simulink model "M10B39"  (R2025a)
settings: Solver=ode23tb  StartTime=0.0  StopTime=20  FixedStep=0.001  MaxStep=0.01  RelTol=1e-3  EnableMultiTasking=on
InitFcn:
  | initAll
values from neighbouring files (symbols this model uses):
  acom = 100    [initAll.m]    (also in initAll_V2.m)
  bcom = 50    [initAll.m]    (also in initAll_V2.m)
  commun = 0*commun    [initAll.m]    (also in initAll_V2.m)
  DataDelay = 0.0*DataDelay    [initAll.m]    (also in initAll_V2.m)
  fB = 50    [initAll.m]    (also in initAll_V2.m)
  Geninit = Generator_init(opdata,SynMach_in_gidx)    [initAll.m]    (also in initAll_V2.m)
  lam = 100    [initAll.m]    (also in initAll_V2.m)
  SgridB = 100    [initAll.m]    (also in initAll_V2.m)
  wB = 2*pi*fB    (= 314.159265359)    [initAll.m]    (also in initAll_V2.m)
undefined symbols (not defined in the file or in its folder): AVm0, c1, c2, c3, c4, c5, c6, cp_nom, ESinit, lambda_nom, P_wind_base, Pelec_base, Pnom, Windinit, YY_load
libraries: spsBistableLib x10, simulink_extras x6, simulink x1
(part 1 of 8)
settings Model: Creator=m  LastModifiedBy=86182
settings SolverCC: AlgebraicLoopSolver=TrustRegion
settings DataIOCC: LimitDataPoints=on  SaveFormat=Array  SignalLoggingSaveFormat=ModelDataLogs  ReturnWorkspaceOutputs=off  SignalLoggingName=sigsOut
settings OptimizationCC: ExpressionDepthLimit=2147483647.0  LifeSpan=inf
settings DebuggingCC: SaveWithParameterizedLinksMsg=none  UnderspecifiedInitializationDetection=Classic  MergeDetectMultiDrivingBlocksExec=none  SignalResolutionControl=TryResolveAllWithWarning  MultiTaskDSMMsg=warning  MultiTaskCondExecSysMsg=none  FcnCallInpInsideContextMsg=warning  UnconnectedInputMsg=warning  UnconnectedOutputMsg=warning  UnconnectedLineMsg=warning  StateNameClashWarn=warning  SFUnexpectedBacktrackingDiag=warning  SFNoUnconditionalDefaultTransitionDiag=warning  SFExecutionAtInitializationDiag=none  ArithmeticOperatorsInVariantConditions=warning
settings HardwareCC: ProdBitPerPointer=32.0  ProdBitPerSizeT=32.0  ProdBitPerPtrDiffT=32.0  ProdLargestAtomicFloat=None  ProdIntDivRoundTo=Undefined  ProdEndianess=Unspecified  ProdWordSize=32.0  ProdHWDeviceType=32-bit Generic  TargetUnknown=on
settings ModelReferenceCC: EnableRefExpFcnMdlSchedulingChecks=on  PropagateSignalLabelsOutOfModel=off
settings SFSimCC: SimUseLocalCustomCode=off  CustomCodeUndefinedFunction=UseInterfaceOnly
settings RTWCC: RTWUseLocalCustomCode=off  GPUComputeCapability=3.5
settings CodeAppCC: StateflowObjectComments=on
settings GRTTargetCC: TargetLangStandard=C89/C90 (ANSI)  CombineOutputUpdateFcns=off  GRTInterface=on
settings ConfigComp: CovMetricSettings=dw  CovSaveCumulativeToWorkspaceVar=on  CovSaveSingleToWorkspaceVar=on  CovExternalEMLEnable=off  CovSFcnEnable=off

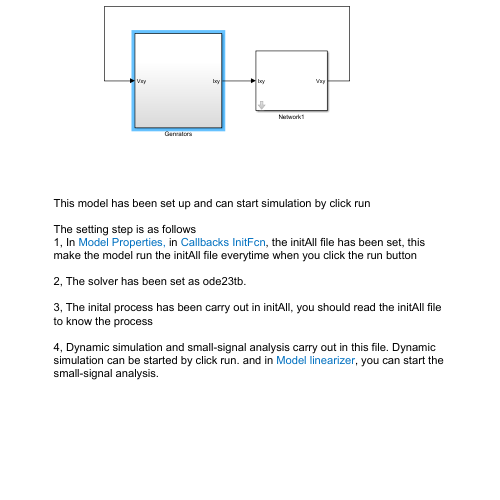
[thumbnail: Simulink's stored preview of the top-level diagram]
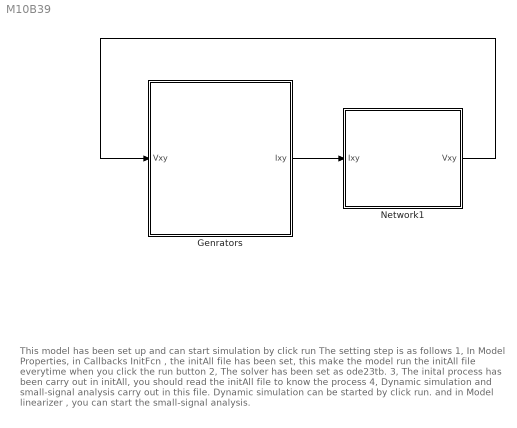
== system M10B39 ==
  note: This model has been set up and can start simulation by click run
      |
      | The setting step is as follows
      | 1, In Model Properties, in Callbacks InitFcn , the initAll file has been set, this make the model run the initAll file everytime when you click the run button
      |
      | 2, The solver has been set as ode23tb.
      |
      | 3, The inital process has been carry out in initAll, you should read the initAll file to know the process
      |
      | 4, Dynamic simulation and small-signal analysis carry out in this file. Dynamic simulation can be started by click run. and in Model linearizer , you can start the small-signal analysis.
  Genrators : Subsystem
  Network1 : Subsystem  mask{YY_load=YY_load, ng=10}
  wires:
  Genrators/1(Ixy) -> Network1/1(Ixy)
  Network1/1(Vxy) -> Genrators/1(Vxy)

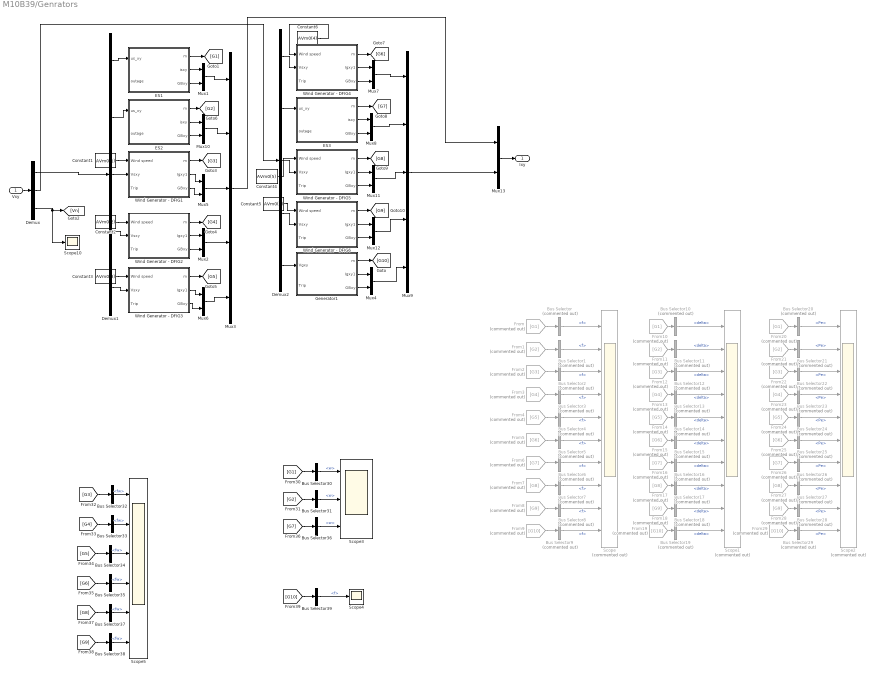
== system M10B39/Genrators ==
  Vxy : Inport
  Bus Selector{,1..9} (10 alike) : BusSelector  Commented=on  OutputSignals=f
  Bus Selector{10..19} (10 alike) : BusSelector  Commented=on  OutputSignals=delta
  Bus Selector{20..29} (10 alike) : BusSelector  Commented=on  OutputSignals=Pe
  Bus Selector30 : BusSelector  OutputSignals=w
  Bus Selector31 : BusSelector  OutputSignals=w
  Bus Selector{32..35,37..38} (6 alike) : BusSelector  OutputSignals=fw
  Bus Selector36 : BusSelector  OutputSignals=w
  Bus Selector39 : BusSelector  OutputSignals=f
  Constant1 : Constant  Value=AVm0(1)
  Constant2 : Constant  Value=AVm0(2)
  Constant3 : Constant  Value=AVm0(3)
  Constant4 : Constant  Value=AVm0(5)
  Constant5 : Constant  Value=AVm0(6)
  Constant6 : Constant  Value=AVm0(4)
  Demux : Demux  Outputs=[10 10 29]
      settings: DisplayOption=none
  Demux1 : Demux  Outputs=5
      settings: DisplayOption=none
  Demux2 : Demux  Outputs=5
      settings: DisplayOption=none
  ES1 : Subsystem  mask{SvscB=ESinit.SvscBi(1), SgridB=SgridB, Kppll_VSC=ESinit.Kppll(1), Kipll_VSC=ESinit.Kipll(1), Dels_hvdc=ESinit.Dels_hvdc(1), Lpr=ESinit.Lpr(1), Rpr=ESinit.Rpr(1), wB=wB, Is_xA_0=ESinit.Isx0(1), Is_yA_0=ESinit.Isy0(1), KpP_VSC_A=ESinit.KpP(1), KiP_VSC_A=ESinit.KiP(1), KpId_VSC_A=ESinit.KpId(1), KiId_VSC_A=ESinit.KiId(1), KpQ_VSC_A=ESinit.KpQ(1), KiQ_VSC_A=ESinit.KiQ(1), KpIq_VSC_A=ESinit.KpIq(1), KiIq_VSC_A=ESinit.KiIq(1), Md_A_0=ESinit.Md0(1), Mq_A_0=ESinit.Mq0(1), Nd_A_0=ESinit.Nd0(1), Nq_A_0=ESinit.Nq0(1), KIR=ESinit.Kir(1), Kdroop=ESinit.Kdroop(1), Kdistributed=ESinit.Kdistributed(1), Kdistributed_d=ESinit.Kdistributed_d(1), Kpac_VSC_A=ESinit.Kpac(1), Kiac_VSC_A=ESinit.Kiac(1), P0=ESinit.P0(1), Q0=ESinit.Q0(1), usd0=ESinit.Usd0(1)}
      mask prompts: Kppll_VSC "Kppll"; Kipll_VSC "Kipll"; KpP_VSC_A "KpP"; KiP_VSC_A "KiP"; KpId_VSC_A "KpId"; KiId_VSC_A "KiId"; KpQ_VSC_A "KpQ"; KiQ_VSC_A "KiQ"; KpIq_VSC_A "KpIq"; KiIq_VSC_A "KiIq"; Kpac_VSC_A "Kpac"; Kiac_VSC_A "Kiac"
      mask DialogControl Container48 Prompt: Base value
      mask DialogControl Container7 Prompt: PLL
      mask DialogControl Container5 Prompt: Control parameter
      mask DialogControl Container8 Prompt: inital value
      mask DialogControl Container9 Prompt: AC side
      mask DialogControl Container10 Prompt: Parameter
      mask DialogControl Container11 Prompt: Initial value
      mask DialogControl Container18 Prompt: Control parameter
      mask DialogControl Container19 Prompt: d_axis_control parameter
      mask DialogControl Container23 Prompt: d_axis_control=1
      mask DialogControl Container26 Prompt: inner current control
      mask DialogControl Container21 Prompt: q_axis_control parameter
      mask DialogControl Container29 Prompt: q_axis_control=1
      mask DialogControl Container31 Prompt: inner current control
      mask DialogControl Container22 Prompt: inital value
      mask DialogControl Container35 Prompt: outer controller
      mask DialogControl Container36 Prompt: inner control
      mask DialogControl Container27 Prompt: Inertia control
      mask DialogControl Container28 Prompt: droop control
      mask DialogControl Container300 Prompt: distributed control
      mask DialogControl Container301 Prompt: Droop distributed control
      mask DialogControl Container40 Prompt: usdq_control
      mask DialogControl Container41 Prompt: PQinitial
      mask DialogControl Container42 Prompt: usd0initial
  ES2 : Subsystem  mask{SvscB=ESinit.SvscBi(2), SgridB=SgridB, Kppll_VSC=ESinit.Kppll(2), Kipll_VSC=ESinit.Kipll(2), Dels_hvdc=ESinit.Dels_hvdc(2), Lpr=ESinit.Lpr(2), Rpr=ESinit.Rpr(2), wB=wB, Is_xA_0=ESinit.Isx0(2), Is_yA_0=ESinit.Isy0(2), KpP_VSC_A=ESinit.KpP(2), KiP_VSC_A=ESinit.KiP(2), KpId_VSC_A=ESinit.KpId(2), KiId_VSC_A=ESinit.KiId(2), KpQ_VSC_A=ESinit.KpQ(2), KiQ_VSC_A=ESinit.KiQ(2), KpIq_VSC_A=ESinit.KpIq(2), KiIq_VSC_A=ESinit.KiIq(2), Md_A_0=ESinit.Md0(2), Mq_A_0=ESinit.Mq0(2), Nd_A_0=ESinit.Nd0(2), Nq_A_0=ESinit.Nq0(2), KIR=ESinit.Kir(2), Kdroop=ESinit.Kdroop(2), Kdistributed=ESinit.Kdistributed(2), Kdistributed_d=ESinit.Kdistributed_d(2), Kpac_VSC_A=ESinit.Kpac(2), Kiac_VSC_A=ESinit.Kiac(2), P0=ESinit.P0(2), Q0=ESinit.Q0(2), usd0=ESinit.Usd0(2)}
      mask prompts: Kppll_VSC "Kppll"; Kipll_VSC "Kipll"; KpP_VSC_A "KpP"; KiP_VSC_A "KiP"; KpId_VSC_A "KpId"; KiId_VSC_A "KiId"; KpQ_VSC_A "KpQ"; KiQ_VSC_A "KiQ"; KpIq_VSC_A "KpIq"; KiIq_VSC_A "KiIq"; Kpac_VSC_A "Kpac"; Kiac_VSC_A "Kiac"
      mask DialogControl Container48 Prompt: Base value
      mask DialogControl Container7 Prompt: PLL
      mask DialogControl Container5 Prompt: Control parameter
      mask DialogControl Container8 Prompt: inital value
      mask DialogControl Container9 Prompt: AC side
      mask DialogControl Container10 Prompt: Parameter
      mask DialogControl Container11 Prompt: Initial value
      mask DialogControl Container18 Prompt: Control parameter
      mask DialogControl Container19 Prompt: d_axis_control parameter
      mask DialogControl Container23 Prompt: d_axis_control=1
      mask DialogControl Container26 Prompt: inner current control
      mask DialogControl Container21 Prompt: q_axis_control parameter
      mask DialogControl Container29 Prompt: q_axis_control=1
      mask DialogControl Container31 Prompt: inner current control
      mask DialogControl Container22 Prompt: inital value
      mask DialogControl Container35 Prompt: outer controller
      mask DialogControl Container36 Prompt: inner control
      mask DialogControl Container27 Prompt: Inertia control
      mask DialogControl Container28 Prompt: droop control
      mask DialogControl Container300 Prompt: distributed control
      mask DialogControl Container301 Prompt: Droop distributed control
      mask DialogControl Container40 Prompt: usdq_control
      mask DialogControl Container41 Prompt: PQinitial
      mask DialogControl Container42 Prompt: usd0initial
  ES3 : Subsystem  mask{SvscB=ESinit.SvscBi(3), SgridB=SgridB, Kppll_VSC=ESinit.Kppll(3), Kipll_VSC=ESinit.Kipll(3), Dels_hvdc=ESinit.Dels_hvdc(3), Lpr=ESinit.Lpr(3), Rpr=ESinit.Rpr(3), wB=wB, Is_xA_0=ESinit.Isx0(3), Is_yA_0=ESinit.Isy0(3), KpP_VSC_A=ESinit.KpP(3), KiP_VSC_A=ESinit.KiP(3), KpId_VSC_A=ESinit.KpId(3), KiId_VSC_A=ESinit.KiId(3), KpQ_VSC_A=ESinit.KpQ(3), KiQ_VSC_A=ESinit.KiQ(3), KpIq_VSC_A=ESinit.KpIq(3), KiIq_VSC_A=ESinit.KiIq(3), Md_A_0=ESinit.Md0(3), Mq_A_0=ESinit.Mq0(3), Nd_A_0=ESinit.Nd0(3), Nq_A_0=ESinit.Nq0(3), KIR=ESinit.Kir(3), Kdroop=ESinit.Kdroop(3), Kdistributed=ESinit.Kdistributed(3), Kdistributed_d=ESinit.Kdistributed_d(3), Kpac_VSC_A=ESinit.Kpac(3), Kiac_VSC_A=ESinit.Kiac(3), P0=ESinit.P0(3), Q0=ESinit.Q0(3), usd0=ESinit.Usd0(3)}
      mask prompts: Kppll_VSC "Kppll"; Kipll_VSC "Kipll"; KpP_VSC_A "KpP"; KiP_VSC_A "KiP"; KpId_VSC_A "KpId"; KiId_VSC_A "KiId"; KpQ_VSC_A "KpQ"; KiQ_VSC_A "KiQ"; KpIq_VSC_A "KpIq"; KiIq_VSC_A "KiIq"; Kpac_VSC_A "Kpac"; Kiac_VSC_A "Kiac"
      mask DialogControl Container48 Prompt: Base value
      mask DialogControl Container7 Prompt: PLL
      mask DialogControl Container5 Prompt: Control parameter
      mask DialogControl Container8 Prompt: inital value
      mask DialogControl Container9 Prompt: AC side
      mask DialogControl Container10 Prompt: Parameter
      mask DialogControl Container11 Prompt: Initial value
      mask DialogControl Container18 Prompt: Control parameter
      mask DialogControl Container19 Prompt: d_axis_control parameter
      mask DialogControl Container23 Prompt: d_axis_control=1
      mask DialogControl Container26 Prompt: inner current control
      mask DialogControl Container21 Prompt: q_axis_control parameter
      mask DialogControl Container29 Prompt: q_axis_control=1
      mask DialogControl Container31 Prompt: inner current control
      mask DialogControl Container22 Prompt: inital value
      mask DialogControl Container35 Prompt: outer controller
      mask DialogControl Container36 Prompt: inner control
      mask DialogControl Container27 Prompt: Inertia control
      mask DialogControl Container28 Prompt: droop control
      mask DialogControl Container300 Prompt: distributed control
      mask DialogControl Container301 Prompt: Droop distributed control
      mask DialogControl Container40 Prompt: usdq_control
      mask DialogControl Container41 Prompt: PQinitial
      mask DialogControl Container42 Prompt: usd0initial
  From : From  Commented=on  GotoTag=G1
  From1 : From  Commented=on  GotoTag=G2
  From10 : From  Commented=on  GotoTag=G1
  From11 : From  Commented=on  GotoTag=G2
  From12 : From  Commented=on  GotoTag=G3
  From13 : From  Commented=on  GotoTag=G4
  From14 : From  Commented=on  GotoTag=G5
  From15 : From  Commented=on  GotoTag=G6
  From16 : From  Commented=on  GotoTag=G7
  From17 : From  Commented=on  GotoTag=G8
  From18 : From  Commented=on  GotoTag=G9
  From19 : From  Commented=on  GotoTag=G10
  From2 : From  Commented=on  GotoTag=G3
  From20 : From  Commented=on  GotoTag=G1
  From21 : From  Commented=on  GotoTag=G2
  From22 : From  Commented=on  GotoTag=G3
  From23 : From  Commented=on  GotoTag=G4
  From24 : From  Commented=on  GotoTag=G5
  From25 : From  Commented=on  GotoTag=G6
  From26 : From  Commented=on  GotoTag=G7
  From27 : From  Commented=on  GotoTag=G8
  From28 : From  Commented=on  GotoTag=G9
  From29 : From  Commented=on  GotoTag=G10
  From3 : From  Commented=on  GotoTag=G4
  From4 : From  Commented=on  GotoTag=G5
  From5 : From  Commented=on  GotoTag=G6
  From6 : From  Commented=on  GotoTag=G7
  From7 : From  Commented=on  GotoTag=G8
  From8 : From  Commented=on  GotoTag=G9
  From9 : From  Commented=on  GotoTag=G10
  Generator1 : Subsystem  mask{wB=wB, SgenB=Geninit.SgenB(1), SgridB=SgridB, Xq=Geninit.Xq(1), Xq1=Geninit.Xq1(1), Xq11=Geninit.Xq11(1), Tq0=Geninit.Tq0(1), Tq10=Geninit.Tq10(1), Eq10=Geninit.Eq1(1), Eq110=Geninit.Eq11(1), Xd=Geninit.Xd(1), Xd1=Geninit.Xd1(1), Xd11=Geninit.Xd11(1), Td0=Geninit.Td0(1), Td10=Geninit.Td10(1), Ed10=Geninit.Ed1(1), Ed110=Geninit.Ed11(1), H=Geninit.Tj(1), D=Geninit.D(1), delta0=Geninit.Delta(1), w0=1, Pm0=Geninit.Pm0(1), Ka=Geninit.Ka(1), Tb=Geninit.Tb(1), Tc=Geninit.Tc(1), Efmax=Geninit.Efmax(1), Efmin=Geninit.Efmin(1), Vref=Geninit.Vref(1), Ef10=Geninit.Vf1(1), S_PSS=Geninit.EnablePSS(1), Kpss=Geninit.kpss(1), Tw_P=Geninit.Tw_P(1), T1_P=Geninit.T1_P(1), T2_P=Geninit.T2_P(1), T3_P=Geninit.T3_P(1), T4_P=Geninit.T4_P(1), Upmax=Geninit.Upmax(1), Upmin=Geninit.Upmin(1), S_Gov=Geninit.Enablegov(1), a_G=Geninit.a_G(1), b_G=Geninit.b_G(1), Tg_G=Geninit.Tg_G(1), dPmax=Geninit.dPmax(1), dPmin=Geninit.dPmin(1)}
      mask prompts: S_PSS "Enable PSS"; Tw_P "Tw"; T1_P "T1"; T2_P "T2"; T3_P "T3"; T4_P "T4"; S_Gov "Enable Governor"; a_G "a"; b_G "b"; Tg_G "Tg"
      mask help: This is a six-order synchronous generator with exciter system, governor and PSS.
      mask DialogControl Container6 Prompt: Machine parameter
      mask DialogControl Container3 Prompt: q axis parameter
      mask DialogControl ParameterGroupVar Prompt: d axis parameter
      mask DialogControl Container4 Prompt: machine parameter
      mask DialogControl Container12 Prompt: Excitation System parameter
      mask DialogControl Container20 Prompt: parameter
      mask DialogControl Container21 Prompt: inital value
      mask DialogControl Container10 Prompt: PSS parameter
      mask DialogControl Container13 Prompt: Governor parameter
  Mux{1..2,4..8,10..13} (11 alike) : Mux  Inputs=2
  Mux3 : Mux  Inputs=5
  Mux9 : Mux  Inputs=5
  Scope : Scope  Commented=on  NumInputPorts=10
      settings: ActiveDisplayYMinimum=0.99999999999963185  ActiveDisplayYMaximum=1.0000000000007851
  Scope1 : Scope  Commented=on  NumInputPorts=10
      settings: ActiveDisplayYMinimum=-0.16939  ActiveDisplayYMaximum=1.28958  DataLoggingVariableName=ScopeData2
  Scope10 : Scope
      settings: ActiveDisplayYMinimum=-247.3342796066861  ActiveDisplayYMaximum=2229.7825782583691  DataLoggingVariableName=ScopeData4
  Scope2 : Scope  Commented=on  NumInputPorts=10
      settings: ActiveDisplayYMinimum=1.62845  ActiveDisplayYMaximum=10.34387  DataLoggingVariableName=ScopeData3
  Scope3 : Scope  NumInputPorts=3
      settings: ActiveDisplayYMinimum=-0.99388665537626475  ActiveDisplayYMaximum=1.3842075167058556  DataLoggingVariableName=ScopeData16
  Scope4 : Scope
      settings: ActiveDisplayYMinimum=0.975520008796966  ActiveDisplayYMaximum=1.0053960624978895  DataLoggingVariableName=ScopeData17
  Scope5 : Scope  NumInputPorts=6
      settings: ActiveDisplayYMinimum=0.99999999999963185  ActiveDisplayYMaximum=1.0000000000007851  DataLoggingVariableName=ScopeData18
  Wind Generator - DFIG1 : Subsystem  mask{NN=Windinit.NN(1), SwgBi=Windinit.SwgBi(1), SmecBi=100, SgridB=SgridB, Atheta=Windinit.Atheta(1), Kppll=Windinit.Kppll_wind(1), Kipll=Windinit.Kipll_wind(1), pitch=[500 45 2], Srotors=1.3, H=Windinit.H(1), Wr0=Windinit.Wr0(1), Xa=Windinit.Xa(1), Xa1=Windinit.Xa1(1), Lm=Windinit.Lm(1), Lr=Windinit.Lr(1), Rs=Windinit.Rs(1), Ls=Windinit.Ls(1), Ta0=Windinit.Ta0(1), NPf=Windinit.NPf(1), Za=Windinit.Za{1}, Ex0=Windinit.Ex_ref(1), Ey0=Windinit.Ey_ref(1), wB=wB, KpP_rw=Windinit.KpP_rw(1), KiP_rw=Windinit.KiP_rw(1), KpId_rw=Windinit.KpId_rw(1), KiId_rw=Windinit.KiId_rw(1), KpQ_rw=Windinit.KpQ_rw(1), KiQ_rw=Windinit.KiQ_rw(1), KpIq_rw=Windinit.KpIq_rw(1), KiIq_rw=Windinit.KiIq_rw(1), Ird_ref=Windinit.Ird_ref(1), Irq_ref=Windinit.Irq_ref(1), Qs0=Windinit.Qs0(1), KpDC_gw=Windinit.KpDC_gw(1), KiDC_gw=Windinit.KiDC_gw(1), KpId_gw=Windinit.KpId_gw(1), KiId_gw=Windinit.KiId_gw(1), KpIq_gw=Windinit.KpIq_gw(1), KiIq_gw=Windinit.KiIq_gw(1), Vdc_w=Windinit.Vdc_w(1), Icd_ref=Windinit.Icd_ref(1), Icq_ref=Windinit.Icq_ref(1), Vcd_ref=Windinit.Vcd_ref(1), Vcq_ref=Windinit.Vcq_ref(1), Lg=Windinit.Lg(1), Rg=Windinit.Rg(1), Icx0=Windinit.Icx0(1), Icy0=Windinit.Icy0(1), C_w=Windinit.C_w(1), Vdc0=Windinit.Vdc0(1)}
      mask prompts: pitch "pitch_gain，pitch_max，pitch_rate"; Srotors "Start Rotor Speed"; Ex0 "Ex"; Ey0 "Ey"
      mask init:
      | pitch_gain=pitch(1);
      | pitch_max=pitch(2);
      | pitch_rate=pitch(3);
      | 
      | %该风机模型的基准容量
      | 
      | SwgeqB=SwgBi.*NN;
      mask DialogControl Container4 Prompt: PLL/Wind turbine
      mask DialogControl Container31 Prompt: Base value
      mask DialogControl Container23 Prompt: PLL
      mask DialogControl Container6 Prompt: inital value
      mask DialogControl Container5 Prompt: PI parameter
      mask DialogControl Container24 Prompt: Wind turbine
      mask DialogControl Container25 Prompt: pitch control
      mask DialogControl Container7 Prompt: Machine parameter
      mask DialogControl Container8 Prompt: Rotor
      mask DialogControl Container9 Prompt: Machine
      mask DialogControl Container10 Prompt: parameter
      mask DialogControl Container11 Prompt: inital value
      mask DialogControl Container12 Prompt: Rotor side control
      mask DialogControl Container13 Prompt: Control parameter
      mask DialogControl Container14 Prompt: Initial value
      mask DialogControl Container15 Prompt: reactive power
      mask DialogControl Container16 Prompt: Grid side control
      mask DialogControl Container17 Prompt: parameter
      mask DialogControl Container18 Prompt: reference
      mask DialogControl Container19 Prompt: inital value
      mask DialogControl Container20 Prompt: converter function
      mask DialogControl Container21 Prompt: inital value
      mask DialogControl Container22 Prompt: DC function
  Wind Generator - DFIG2 : Subsystem  mask{NN=Windinit.NN(2), SwgBi=Windinit.SwgBi(2), SmecBi=100, SgridB=SgridB, Atheta=Windinit.Atheta(2), Kppll=Windinit.Kppll_wind(2), Kipll=Windinit.Kipll_wind(2), pitch=[500 45 2], Srotors=1.3, H=Windinit.H(2), Wr0=Windinit.Wr0(2), Xa=Windinit.Xa(2), Xa1=Windinit.Xa1(2), Lm=Windinit.Lm(2), Lr=Windinit.Lr(2), Rs=Windinit.Rs(2), Ls=Windinit.Ls(2), Ta0=Windinit.Ta0(2), NPf=Windinit.NPf(2), Za=Windinit.Za{2}, Ex0=Windinit.Ex_ref(2), Ey0=Windinit.Ey_ref(2), wB=wB, KpP_rw=Windinit.KpP_rw(2), KiP_rw=Windinit.KiP_rw(2), KpId_rw=Windinit.KpId_rw(2), KiId_rw=Windinit.KiId_rw(2), KpQ_rw=Windinit.KpQ_rw(2), KiQ_rw=Windinit.KiQ_rw(2), KpIq_rw=Windinit.KpIq_rw(2), KiIq_rw=Windinit.KiIq_rw(2), Ird_ref=Windinit.Ird_ref(2), Irq_ref=Windinit.Irq_ref(2), Qs0=Windinit.Qs0(2), KpDC_gw=Windinit.KpDC_gw(2), KiDC_gw=Windinit.KiDC_gw(2), KpId_gw=Windinit.KpId_gw(2), KiId_gw=Windinit.KiId_gw(2), KpIq_gw=Windinit.KpIq_gw(2), KiIq_gw=Windinit.KiIq_gw(2), Vdc_w=Windinit.Vdc_w(2), Icd_ref=Windinit.Icd_ref(2), Icq_ref=Windinit.Icq_ref(2), Vcd_ref=Windinit.Vcd_ref(2), Vcq_ref=Windinit.Vcq_ref(2), Lg=Windinit.Lg(2), Rg=Windinit.Rg(2), Icx0=Windinit.Icx0(2), Icy0=Windinit.Icy0(2), C_w=Windinit.C_w(2), Vdc0=Windinit.Vdc0(2)}
      mask prompts: pitch "pitch_gain，pitch_max，pitch_rate"; Srotors "Start Rotor Speed"; Ex0 "Ex"; Ey0 "Ey"
      mask init:
      | pitch_gain=pitch(1);
      | pitch_max=pitch(2);
      | pitch_rate=pitch(3);
      | 
      | %该风机模型的基准容量
      | 
      | SwgeqB=SwgBi.*NN;
      mask DialogControl Container4 Prompt: PLL/Wind turbine
      mask DialogControl Container31 Prompt: Base value
      mask DialogControl Container23 Prompt: PLL
      mask DialogControl Container6 Prompt: inital value
      mask DialogControl Container5 Prompt: PI parameter
      mask DialogControl Container24 Prompt: Wind turbine
      mask DialogControl Container25 Prompt: pitch control
      mask DialogControl Container7 Prompt: Machine parameter
      mask DialogControl Container8 Prompt: Rotor
      mask DialogControl Container9 Prompt: Machine
      mask DialogControl Container10 Prompt: parameter
      mask DialogControl Container11 Prompt: inital value
      mask DialogControl Container12 Prompt: Rotor side control
      mask DialogControl Container13 Prompt: Control parameter
      mask DialogControl Container14 Prompt: Initial value
      mask DialogControl Container15 Prompt: reactive power
      mask DialogControl Container16 Prompt: Grid side control
      mask DialogControl Container17 Prompt: parameter
      mask DialogControl Container18 Prompt: reference
      mask DialogControl Container19 Prompt: inital value
      mask DialogControl Container20 Prompt: converter function
      mask DialogControl Container21 Prompt: inital value
      mask DialogControl Container22 Prompt: DC function
  Wind Generator - DFIG3 : Subsystem  mask{NN=Windinit.NN(3), SwgBi=Windinit.SwgBi(3), SmecBi=100, SgridB=SgridB, Atheta=Windinit.Atheta(3), Kppll=Windinit.Kppll_wind(3), Kipll=Windinit.Kipll_wind(3), pitch=[500 45 2], Srotors=1.3, H=Windinit.H(3), Wr0=Windinit.Wr0(3), Xa=Windinit.Xa(3), Xa1=Windinit.Xa1(3), Lm=Windinit.Lm(3), Lr=Windinit.Lr(3), Rs=Windinit.Rs(3), Ls=Windinit.Ls(3), Ta0=Windinit.Ta0(3), NPf=Windinit.NPf(3), Za=Windinit.Za{3}, Ex0=Windinit.Ex_ref(3), Ey0=Windinit.Ey_ref(3), wB=wB, KpP_rw=Windinit.KpP_rw(3), KiP_rw=Windinit.KiP_rw(3), KpId_rw=Windinit.KpId_rw(3), KiId_rw=Windinit.KiId_rw(3), KpQ_rw=Windinit.KpQ_rw(3), KiQ_rw=Windinit.KiQ_rw(3), KpIq_rw=Windinit.KpIq_rw(3), KiIq_rw=Windinit.KiIq_rw(3), Ird_ref=Windinit.Ird_ref(3), Irq_ref=Windinit.Irq_ref(3), Qs0=Windinit.Qs0(3), KpDC_gw=Windinit.KpDC_gw(3), KiDC_gw=Windinit.KiDC_gw(3), KpId_gw=Windinit.KpId_gw(3), KiId_gw=Windinit.KiId_gw(3), KpIq_gw=Windinit.KpIq_gw(3), KiIq_gw=Windinit.KiIq_gw(2), Vdc_w=Windinit.Vdc_w(3), Icd_ref=Windinit.Icd_ref(3), Icq_ref=Windinit.Icq_ref(3), Vcd_ref=Windinit.Vcd_ref(3), Vcq_ref=Windinit.Vcq_ref(3), Lg=Windinit.Lg(3), Rg=Windinit.Rg(3), Icx0=Windinit.Icx0(3), Icy0=Windinit.Icy0(3), C_w=Windinit.C_w(3), Vdc0=Windinit.Vdc0(3)}
      mask prompts: pitch "pitch_gain，pitch_max，pitch_rate"; Srotors "Start Rotor Speed"; Ex0 "Ex"; Ey0 "Ey"
      mask init:
      | pitch_gain=pitch(1);
      | pitch_max=pitch(2);
      | pitch_rate=pitch(3);
      | 
      | %该风机模型的基准容量
      | 
      | SwgeqB=SwgBi.*NN;
      mask DialogControl Container4 Prompt: PLL/Wind turbine
      mask DialogControl Container31 Prompt: Base value
      mask DialogControl Container23 Prompt: PLL
      mask DialogControl Container6 Prompt: inital value
      mask DialogControl Container5 Prompt: PI parameter
      mask DialogControl Container24 Prompt: Wind turbine
      mask DialogControl Container25 Prompt: pitch control
      mask DialogControl Container7 Prompt: Machine parameter
      mask DialogControl Container8 Prompt: Rotor
      mask DialogControl Container9 Prompt: Machine
      mask DialogControl Container10 Prompt: parameter
      mask DialogControl Container11 Prompt: inital value
      mask DialogControl Container12 Prompt: Rotor side control
      mask DialogControl Container13 Prompt: Control parameter
      mask DialogControl Container14 Prompt: Initial value
      mask DialogControl Container15 Prompt: reactive power
      mask DialogControl Container16 Prompt: Grid side control
      mask DialogControl Container17 Prompt: parameter
      mask DialogControl Container18 Prompt: reference
      mask DialogControl Container19 Prompt: inital value
      mask DialogControl Container20 Prompt: converter function
      mask DialogControl Container21 Prompt: inital value
      mask DialogControl Container22 Prompt: DC function
  Wind Generator - DFIG4 : Subsystem  mask{NN=Windinit.NN(4), SwgBi=Windinit.SwgBi(4), SmecBi=100, SgridB=SgridB, Atheta=Windinit.Atheta(4), Kppll=Windinit.Kppll_wind(4), Kipll=Windinit.Kipll_wind(4), pitch=[500 45 2], Srotors=1.3, H=Windinit.H(4), Wr0=Windinit.Wr0(4), Xa=Windinit.Xa(4), Xa1=Windinit.Xa1(4), Lm=Windinit.Lm(4), Lr=Windinit.Lr(4), Rs=Windinit.Rs(4), Ls=Windinit.Ls(4), Ta0=Windinit.Ta0(4), NPf=Windinit.NPf(4), Za=Windinit.Za{4}, Ex0=Windinit.Ex_ref(4), Ey0=Windinit.Ey_ref(4), wB=wB, KpP_rw=Windinit.KpP_rw(4), KiP_rw=Windinit.KiP_rw(4), KpId_rw=Windinit.KpId_rw(4), KiId_rw=Windinit.KiId_rw(4), KpQ_rw=Windinit.KpQ_rw(4), KiQ_rw=Windinit.KiQ_rw(4), KpIq_rw=Windinit.KpIq_rw(4), KiIq_rw=Windinit.KiIq_rw(4), Ird_ref=Windinit.Ird_ref(4), Irq_ref=Windinit.Irq_ref(4), Qs0=Windinit.Qs0(4), KpDC_gw=Windinit.KpDC_gw(4), KiDC_gw=Windinit.KiDC_gw(4), KpId_gw=Windinit.KpId_gw(4), KiId_gw=Windinit.KiId_gw(4), KpIq_gw=Windinit.KpIq_gw(4), KiIq_gw=Windinit.KiIq_gw(4), Vdc_w=Windinit.Vdc_w(4), Icd_ref=Windinit.Icd_ref(4), Icq_ref=Windinit.Icq_ref(4), Vcd_ref=Windinit.Vcd_ref(4), Vcq_ref=Windinit.Vcq_ref(4), Lg=Windinit.Lg(4), Rg=Windinit.Rg(4), Icx0=Windinit.Icx0(4), Icy0=Windinit.Icy0(4), C_w=Windinit.C_w(4), Vdc0=Windinit.Vdc0(4)}
      mask prompts: pitch "pitch_gain，pitch_max，pitch_rate"; Srotors "Start Rotor Speed"; Ex0 "Ex"; Ey0 "Ey"
      mask init:
      | pitch_gain=pitch(1);
      | pitch_max=pitch(2);
      | pitch_rate=pitch(3);
      | 
      | %该风机模型的基准容量
      | 
      | SwgeqB=SwgBi.*NN;
      mask DialogControl Container4 Prompt: PLL/Wind turbine
      mask DialogControl Container31 Prompt: Base value
      mask DialogControl Container23 Prompt: PLL
      mask DialogControl Container6 Prompt: inital value
      mask DialogControl Container5 Prompt: PI parameter
      mask DialogControl Container24 Prompt: Wind turbine
      mask DialogControl Container25 Prompt: pitch control
      mask DialogControl Container7 Prompt: Machine parameter
      mask DialogControl Container8 Prompt: Rotor
      mask DialogControl Container9 Prompt: Machine
      mask DialogControl Container10 Prompt: parameter
      mask DialogControl Container11 Prompt: inital value
      mask DialogControl Container12 Prompt: Rotor side control
      mask DialogControl Container13 Prompt: Control parameter
      mask DialogControl Container14 Prompt: Initial value
      mask DialogControl Container15 Prompt: reactive power
      mask DialogControl Container16 Prompt: Grid side control
      mask DialogControl Container17 Prompt: parameter
      mask DialogControl Container18 Prompt: reference
      mask DialogControl Container19 Prompt: inital value
      mask DialogControl Container20 Prompt: converter function
      mask DialogControl Container21 Prompt: inital value
      mask DialogControl Container22 Prompt: DC function
  Wind Generator - DFIG5 : Subsystem  mask{NN=Windinit.NN(5), SwgBi=Windinit.SwgBi(5), SmecBi=100, SgridB=SgridB, Atheta=Windinit.Atheta(5), Kppll=Windinit.Kppll_wind(5), Kipll=Windinit.Kipll_wind(5), pitch=[500 45 2], Srotors=1.3, H=Windinit.H(5), Wr0=Windinit.Wr0(5), Xa=Windinit.Xa(5), Xa1=Windinit.Xa1(5), Lm=Windinit.Lm(5), Lr=Windinit.Lr(5), Rs=Windinit.Rs(5), Ls=Windinit.Ls(5), Ta0=Windinit.Ta0(5), NPf=Windinit.NPf(5), Za=Windinit.Za{5}, Ex0=Windinit.Ex_ref(5), Ey0=Windinit.Ey_ref(5), wB=wB, KpP_rw=Windinit.KpP_rw(5), KiP_rw=Windinit.KiP_rw(5), KpId_rw=Windinit.KpId_rw(5), KiId_rw=Windinit.KiId_rw(5), KpQ_rw=Windinit.KpQ_rw(5), KiQ_rw=Windinit.KiQ_rw(5), KpIq_rw=Windinit.KpIq_rw(5), KiIq_rw=Windinit.KiIq_rw(5), Ird_ref=Windinit.Ird_ref(5), Irq_ref=Windinit.Irq_ref(5), Qs0=Windinit.Qs0(5), KpDC_gw=Windinit.KpDC_gw(5), KiDC_gw=Windinit.KiDC_gw(5), KpId_gw=Windinit.KpId_gw(5), KiId_gw=Windinit.KiId_gw(5), KpIq_gw=Windinit.KpIq_gw(5), KiIq_gw=Windinit.KiIq_gw(5), Vdc_w=Windinit.Vdc_w(5), Icd_ref=Windinit.Icd_ref(5), Icq_ref=Windinit.Icq_ref(5), Vcd_ref=Windinit.Vcd_ref(5), Vcq_ref=Windinit.Vcq_ref(5), Lg=Windinit.Lg(5), Rg=Windinit.Rg(5), Icx0=Windinit.Icx0(5), Icy0=Windinit.Icy0(5), C_w=Windinit.C_w(5), Vdc0=Windinit.Vdc0(5)}
      mask prompts: pitch "pitch_gain，pitch_max，pitch_rate"; Srotors "Start Rotor Speed"; Ex0 "Ex"; Ey0 "Ey"
      mask init:
      | pitch_gain=pitch(1);
      | pitch_max=pitch(2);
      | pitch_rate=pitch(3);
      | 
      | %该风机模型的基准容量
      | 
      | SwgeqB=SwgBi.*NN;
      mask DialogControl Container4 Prompt: PLL/Wind turbine
      mask DialogControl Container31 Prompt: Base value
      mask DialogControl Container23 Prompt: PLL
      mask DialogControl Container6 Prompt: inital value
      mask DialogControl Container5 Prompt: PI parameter
      mask DialogControl Container24 Prompt: Wind turbine
      mask DialogControl Container25 Prompt: pitch control
      mask DialogControl Container7 Prompt: Machine parameter
      mask DialogControl Container8 Prompt: Rotor
      mask DialogControl Container9 Prompt: Machine
      mask DialogControl Container10 Prompt: parameter
      mask DialogControl Container11 Prompt: inital value
      mask DialogControl Container12 Prompt: Rotor side control
      mask DialogControl Container13 Prompt: Control parameter
      mask DialogControl Container14 Prompt: Initial value
      mask DialogControl Container15 Prompt: reactive power
      mask DialogControl Container16 Prompt: Grid side control
      mask DialogControl Container17 Prompt: parameter
      mask DialogControl Container18 Prompt: reference
      mask DialogControl Container19 Prompt: inital value
      mask DialogControl Container20 Prompt: converter function
      mask DialogControl Container21 Prompt: inital value
      mask DialogControl Container22 Prompt: DC function
  Wind Generator - DFIG6 : Subsystem  mask{NN=Windinit.NN(6), SwgBi=Windinit.SwgBi(6), SmecBi=100, SgridB=SgridB, Atheta=Windinit.Atheta(6), Kppll=Windinit.Kppll_wind(6), Kipll=Windinit.Kipll_wind(6), pitch=[500 45 2], Srotors=1.3, H=Windinit.H(6), Wr0=Windinit.Wr0(6), Xa=Windinit.Xa(6), Xa1=Windinit.Xa1(6), Lm=Windinit.Lm(6), Lr=Windinit.Lr(6), Rs=Windinit.Rs(6), Ls=Windinit.Ls(6), Ta0=Windinit.Ta0(6), NPf=Windinit.NPf(6), Za=Windinit.Za{6}, Ex0=Windinit.Ex_ref(6), Ey0=Windinit.Ey_ref(6), wB=wB, KpP_rw=Windinit.KpP_rw(6), KiP_rw=Windinit.KiP_rw(6), KpId_rw=Windinit.KpId_rw(6), KiId_rw=Windinit.KiId_rw(6), KpQ_rw=Windinit.KpQ_rw(6), KiQ_rw=Windinit.KiQ_rw(6), KpIq_rw=Windinit.KpIq_rw(6), KiIq_rw=Windinit.KiIq_rw(6), Ird_ref=Windinit.Ird_ref(6), Irq_ref=Windinit.Irq_ref(6), Qs0=Windinit.Qs0(6), KpDC_gw=Windinit.KpDC_gw(6), KiDC_gw=Windinit.KiDC_gw(6), KpId_gw=Windinit.KpId_gw(6), KiId_gw=Windinit.KiId_gw(6), KpIq_gw=Windinit.KpIq_gw(6), KiIq_gw=Windinit.KiIq_gw(6), Vdc_w=Windinit.Vdc_w(6), Icd_ref=Windinit.Icd_ref(6), Icq_ref=Windinit.Icq_ref(6), Vcd_ref=Windinit.Vcd_ref(6), Vcq_ref=Windinit.Vcq_ref(6), Lg=Windinit.Lg(6), Rg=Windinit.Rg(6), Icx0=Windinit.Icx0(6), Icy0=Windinit.Icy0(6), C_w=Windinit.C_w(6), Vdc0=Windinit.Vdc0(6)}
      mask prompts: pitch "pitch_gain，pitch_max，pitch_rate"; Srotors "Start Rotor Speed"; Ex0 "Ex"; Ey0 "Ey"
      mask init:
      | pitch_gain=pitch(1);
      | pitch_max=pitch(2);
      | pitch_rate=pitch(3);
      | 
      | %该风机模型的基准容量
      | 
      | SwgeqB=SwgBi.*NN;
      mask DialogControl Container4 Prompt: PLL/Wind turbine
      mask DialogControl Container31 Prompt: Base value
      mask DialogControl Container23 Prompt: PLL
      mask DialogControl Container6 Prompt: inital value
      mask DialogControl Container5 Prompt: PI parameter
      mask DialogControl Container24 Prompt: Wind turbine
      mask DialogControl Container25 Prompt: pitch control
      mask DialogControl Container7 Prompt: Machine parameter
      mask DialogControl Container8 Prompt: Rotor
      mask DialogControl Container9 Prompt: Machine
      mask DialogControl Container10 Prompt: parameter
      mask DialogControl Container11 Prompt: inital value
      mask DialogControl Container12 Prompt: Rotor side control
      mask DialogControl Container13 Prompt: Control parameter
      mask DialogControl Container14 Prompt: Initial value
      mask DialogControl Container15 Prompt: reactive power
      mask DialogControl Container16 Prompt: Grid side control
      mask DialogControl Container17 Prompt: parameter
      mask DialogControl Container18 Prompt: reference
      mask DialogControl Container19 Prompt: inital value
      mask DialogControl Container20 Prompt: converter function
      mask DialogControl Container21 Prompt: inital value
      mask DialogControl Container22 Prompt: DC function
  Ixy : Outport
  wires:
  Mux13/1 -> Ixy/1
  Mux9/1 -> Mux13/2
  Mux3/1 -> Mux13/1
  Vxy/1 -> Demux/1
  Demux/1 -> Demux1/1
  Demux/2 -> Demux2/1
  Demux/3 -> [Vn], Scope10/1
  From/1 -> Bus Selector/1
  From1/1 -> Bus Selector1/1
  From2/1 -> Bus Selector2/1
  From3/1 -> Bus Selector3/1
  From4/1 -> Bus Selector4/1
  From5/1 -> Bus Selector5/1
  From6/1 -> Bus Selector6/1
  From7/1 -> Bus Selector7/1
  From8/1 -> Bus Selector8/1
  From9/1 -> Bus Selector9/1
  Bus Selector/1 -> Scope/1  "<f>"
  Bus Selector1/1 -> Scope/2  "<f>"
  Bus Selector2/1 -> Scope/3  "<f>"
  Bus Selector3/1 -> Scope/4  "<f>"
  Bus Selector4/1 -> Scope/5  "<f>"
  Bus Selector5/1 -> Scope/6  "<f>"
  Bus Selector6/1 -> Scope/7  "<f>"
  Bus Selector7/1 -> Scope/8  "<f>"
  Bus Selector8/1 -> Scope/9  "<f>"
  Bus Selector9/1 -> Scope/10  "<f>"
  From10/1 -> Bus Selector10/1
  From11/1 -> Bus Selector11/1
  From12/1 -> Bus Selector12/1
  From13/1 -> Bus Selector13/1
  From14/1 -> Bus Selector14/1
  From15/1 -> Bus Selector15/1
  From16/1 -> Bus Selector16/1
  From17/1 -> Bus Selector17/1
  From18/1 -> Bus Selector18/1
  From19/1 -> Bus Selector19/1
  Bus Selector19/1 -> Scope1/10  "<delta>"
  Bus Selector18/1 -> Scope1/9  "<delta>"
  Bus Selector17/1 -> Scope1/8  "<delta>"
  Bus Selector16/1 -> Scope1/7  "<delta>"
  Bus Selector15/1 -> Scope1/6  "<delta>"
  Bus Selector14/1 -> Scope1/5  "<delta>"
  Bus Selector13/1 -> Scope1/4  "<delta>"
  Bus Selector12/1 -> Scope1/3  "<delta>"
  Bus Selector11/1 -> Scope1/2  "<delta>"
  Bus Selector10/1 -> Scope1/1  "<delta>"
  From27/1 -> Bus Selector27/1
  From20/1 -> Bus Selector20/1
  From21/1 -> Bus Selector21/1
  From26/1 -> Bus Selector26/1
  From29/1 -> Bus Selector29/1
  From28/1 -> Bus Selector28/1
  From23/1 -> Bus Selector23/1
  From22/1 -> Bus Selector22/1
  From25/1 -> Bus Selector25/1
  From24/1 -> Bus Selector24/1
  Bus Selector20/1 -> Scope2/1  "<Pe>"
  Bus Selector21/1 -> Scope2/2  "<Pe>"
  Bus Selector22/1 -> Scope2/3  "<Pe>"
  Bus Selector23/1 -> Scope2/4  "<Pe>"
  Bus Selector24/1 -> Scope2/5  "<Pe>"
  Bus Selector25/1 -> Scope2/6  "<Pe>"
  Bus Selector26/1 -> Scope2/7  "<Pe>"
  Bus Selector27/1 -> Scope2/8  "<Pe>"
  Bus Selector28/1 -> Scope2/9  "<Pe>"
  Bus Selector29/1 -> Scope2/10  "<Pe>"
  Generator1/1(m) -> [G10]
  Mux4/1 -> Mux9/5
  Generator1/3(GBxy) -> Mux4/2
  Generator1/2(Igxy1) -> Mux4/1
  ES1/1(m) -> [G1]
  Demux1/1 -> ES1/1(us_xy)
  ES1/3(GBxy) -> Mux1/2
  ES1/2(isxy) -> Mux1/1
  Mux1/1 -> Mux3/1
  ES2/2(isxy) -> Mux10/1
  ES2/1(m) -> [G2]
  ES2/3(GBxy) -> Mux10/2
  Mux10/1 -> Mux3/2
  Demux1/2 -> ES2/1(us_xy)
  Wind Generator - DFIG2/3(GBxy) -> Mux2/2
  Wind Generator - DFIG1/2(Igxy1) -> Mux5/1
  Mux2/1 -> Mux3/4
  Wind Generator - DFIG1/1(m) -> [G3]
  Wind Generator - DFIG2/2(Igxy1) -> Mux2/1
  Mux5/1 -> Mux3/3
  Wind Generator - DFIG2/1(m) -> [G4]
  Wind Generator - DFIG1/3(GBxy) -> Mux5/2
  Wind Generator - DFIG3/3(GBxy) -> Mux6/2
  Wind Generator - DFIG3/2(Igxy1) -> Mux6/1
  Wind Generator - DFIG3/1(m) -> [G5]
  Mux6/1 -> Mux3/5
  Demux1/3 -> Wind Generator - DFIG1/2(Vsxy)
  Demux1/4 -> Wind Generator - DFIG2/2(Vsxy)
  Demux1/5 -> Wind Generator - DFIG3/2(Vsxy)
  Wind Generator - DFIG4/3(GBxy) -> Mux7/2
  Wind Generator - DFIG4/2(Igxy1) -> Mux7/1
  Wind Generator - DFIG4/1(m) -> [G6]
  Mux7/1 -> Mux9/1
  Demux2/1 -> Wind Generator - DFIG4/2(Vsxy)
  ES3/2(isxy) -> Mux8/1
  ES3/1(m) -> [G7]
  ES3/3(GBxy) -> Mux8/2
  Mux8/1 -> Mux9/2
  Demux2/2 -> ES3/1(us_xy)
  Wind Generator - DFIG5/1(m) -> [G8]
  Wind Generator - DFIG5/2(Igxy1) -> Mux11/1
  Wind Generator - DFIG5/3(GBxy) -> Mux11/2
  Demux2/3 -> Wind Generator - DFIG5/2(Vsxy)
  Mux11/1 -> Mux9/3
  Demux2/5 -> Generator1/1(Vgxy)
  Wind Generator - DFIG6/1(m) -> [G9]
  Wind Generator - DFIG6/2(Igxy1) -> Mux12/1
  Wind Generator - DFIG6/3(GBxy) -> Mux12/2
  Mux12/1 -> Mux9/4
  Demux2/4 -> Wind Generator - DFIG6/2(Vsxy)
  [G7] -> Bus Selector36/1
  [G10] -> Bus Selector39/1
  [G5] -> Bus Selector34/1
  [G6] -> Bus Selector35/1
  [G9] -> Bus Selector38/1
  [G4] -> Bus Selector33/1
  [G8] -> Bus Selector37/1
  [G2] -> Bus Selector31/1
  [G1] -> Bus Selector30/1
  [G3] -> Bus Selector32/1
  Bus Selector30/1 -> Scope3/1  "<w>"
  Bus Selector31/1 -> Scope3/2  "<w>"
  Bus Selector36/1 -> Scope3/3  "<w>"
  Bus Selector39/1 -> Scope4/1  "<f>"
  Bus Selector32/1 -> Scope5/1  "<fw>"
  Bus Selector33/1 -> Scope5/2  "<fw>"
  Bus Selector34/1 -> Scope5/3  "<fw>"
  Bus Selector35/1 -> Scope5/4  "<fw>"
  Bus Selector38/1 -> Scope5/6  "<fw>"
  Bus Selector37/1 -> Scope5/5  "<fw>"
  Constant1/1 -> Wind Generator - DFIG1/1(Wind speed)
  Constant2/1 -> Wind Generator - DFIG2/1(Wind speed)
  Constant3/1 -> Wind Generator - DFIG3/1(Wind speed)
  Constant4/1 -> Wind Generator - DFIG5/1(Wind speed)
  Constant5/1 -> Wind Generator - DFIG6/1(Wind speed)
  Constant6/1 -> Wind Generator - DFIG4/1(Wind speed)

== system M10B39/Network1 ==
  Ixy : Inport
  Clock : Clock
  Mux : Mux  Inputs=2
  S-Function : S-Function  FunctionName=TS_net_1_new  Parameters=YY_load,ng  SFunctionDeploymentMode=off  EnableBusSupport=off
  S-Function Examples : simulink/User-Defined Functions/S-Function Examples  Commented=on
  S-Function1 : S-Function  Commented=on  Parameters=YY_load,ng  SFunctionDeploymentMode=off  EnableBusSupport=off
  Vxy : Outport
  wires:
  Clock/1 -> Mux/1
  Ixy/1 -> Mux/2
  Mux/1 -> S-Function/1
  S-Function/1 -> Vxy/1

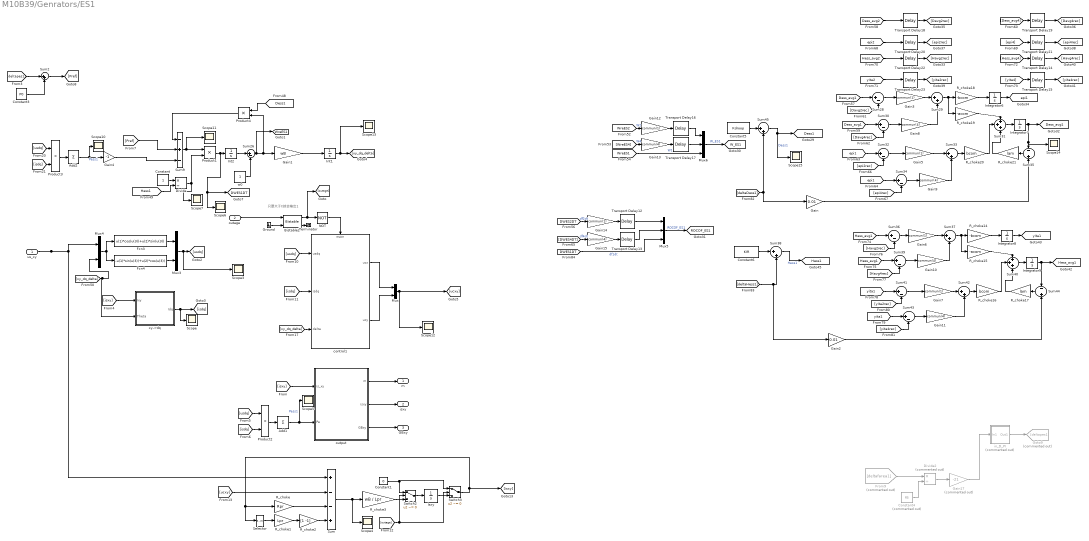
== system M10B39/Genrators/ES1 ==
  note: 只要大于0就会输出1
  us_xy : Inport
  outage : Inport  Port=2
  " control1" : Subsystem
  Add1 : Sum  Inputs=+
  Add2 : Sum  Inputs=+
  Bistable2 : spsBistableLib/Bistable  Qpriority=Set  ic=0  Ts=0
  Constant : Constant
  Constant1 : Constant  Value=0
  Constant3 : Constant  Value=P0
  Constant4 : Constant  Commented=on  Value=fB
  Constant5 : Constant  Value=Kdroop
  Constant6 : Constant  Value=KIR
  Divide : Product  Inputs=*/
  Divide2 : Product  Commented=on  Inputs=*/
  Fcn3 : Fcn  Expr=u(1)*cos(u(3))+u(2)*sin(u(3))
  Fcn4 : Fcn  Expr=-u(1)*sin(u(3))+u(2)*cos(u(3))
  From9 : From  Commented=on  GotoTag=deltafarea1  TagVisibility=global
  Gain : Gain  Gain=0.01
  Gain1 : Gain  Gain=wB  SaturateOnIntegerOverflow=on  OutDataTypeStr=Inherit: Same as input  ParamDataTypeStr=Inherit: Same as input
  Gain{8..11,13,15} (6 alike) : Gain  Gain=commun(4)
  Gain{3,5..7,12,14} (6 alike) : Gain  Gain=commun(1)
  Gain17 : Gain  Commented=on  Gain=-21
  Gain2 : Gain  Gain=0.01
  Gain4 : Gain  Gain=-1
  Goto9 : Goto  Commented=on  GotoTag=deltapes1
  Ground : Ground
  Int1 : Integrator  InitialCondition=Dels_hvdc
  Int2 : Integrator  InitialCondition=1
  Integrator{6..9} (4 alike) : Integrator
  Isxy : Integrator  InitialCondition=[Is_xA_0 Is_yA_0]
  Mux : Mux  Inputs=2
  Mux3 : Mux  Inputs=2
  Mux4 : Mux  Inputs=2
  Mux5 : Mux  Inputs=3
  Mux6 : Mux  Inputs=3
  NOT : Logic  Operator=NOT  AllPortsSameDT=off  OutDataTypeStr=boolean
  Product1 : Product
  Product2 : Product  RndMeth=Zero
  Product3 : Product  RndMeth=Zero
  Product4 : Product
  R_choke : Gain  Gain=Rpr  SaturateOnIntegerOverflow=on  OutDataTypeStr=Inherit: Same as input  ParamDataTypeStr=Inherit: Same as input
  R_choke1 : Gain  Gain=Lpr  SaturateOnIntegerOverflow=on  OutDataTypeStr=Inherit: Same as input  ParamDataTypeStr=Inherit: Same as input
  R_choke14 : Gain  Gain=-bcom  SaturateOnIntegerOverflow=on  OutDataTypeStr=Inherit: Same as input  ParamDataTypeStr=Inherit: Same as input
  R_choke15 : Gain  Gain=-acom  SaturateOnIntegerOverflow=on  OutDataTypeStr=Inherit: Same as input  ParamDataTypeStr=Inherit: Same as input
  R_choke16 : Gain  Gain=bcom  SaturateOnIntegerOverflow=on  OutDataTypeStr=Inherit: Same as input  ParamDataTypeStr=Inherit: Same as input
  R_choke17 : Gain  Gain=lam  SaturateOnIntegerOverflow=on  OutDataTypeStr=Inherit: Same as input  ParamDataTypeStr=Inherit: Same as input
  R_choke18 : Gain  Gain=-bcom  SaturateOnIntegerOverflow=on  OutDataTypeStr=Inherit: Same as input  ParamDataTypeStr=Inherit: Same as input
  R_choke19 : Gain  Gain=-acom  SaturateOnIntegerOverflow=on  OutDataTypeStr=Inherit: Same as input  ParamDataTypeStr=Inherit: Same as input
  R_choke2 : Gain  Gain=[1 -1]  SaturateOnIntegerOverflow=on  OutDataTypeStr=Inherit: Same as input  ParamDataTypeStr=Inherit: Same as input
  R_choke20 : Gain  Gain=bcom  SaturateOnIntegerOverflow=on  OutDataTypeStr=Inherit: Same as input  ParamDataTypeStr=Inherit: Same as input
  R_choke21 : Gain  Gain=lam  SaturateOnIntegerOverflow=on  OutDataTypeStr=Inherit: Same as input  ParamDataTypeStr=Inherit: Same as input
  R_choke3 : Gain  Gain=wB / Lpr  SaturateOnIntegerOverflow=on  OutDataTypeStr=Inherit: Same as input  ParamDataTypeStr=Inherit: Same as input
  Scope{,3..7,10..15} (12 alike) : Scope
      Scope settings: ActiveDisplayYMinimum=-0.0194  ActiveDisplayYMaximum=0.04689
      Scope10 settings: ActiveDisplayYMinimum=-0.6053  ActiveDisplayYMaximum=0.06726
      Scope11 settings: ActiveDisplayYMinimum=-0.1125  ActiveDisplayYMaximum=0.0125  DataLoggingVariableName=ScopeData2
      Scope12 settings: ActiveDisplayYMinimum=0.46883  ActiveDisplayYMaximum=1.25548  DataLoggingVariableName=ScopeData3
      Scope13 settings: ActiveDisplayYMinimum=-4.33823  ActiveDisplayYMaximum=0.36599  DataLoggingVariableName=ScopeData4
      Scope14 settings: ActiveDisplayYMinimum=-0.0418  ActiveDisplayYMaximum=0.37621  DataLoggingVariableName=ScopeData2
      Scope15 settings: ActiveDisplayYMinimum=-1  ActiveDisplayYMaximum=1  DataLoggingVariableName=ScopeData3
      Scope3 settings: ActiveDisplayYMinimum=-0.14332  ActiveDisplayYMaximum=1.14443
      Scope4 settings: ActiveDisplayYMinimum=-2.8E-5  ActiveDisplayYMaximum=2.4E-5  DataLoggingVariableName=ScopeData5
      Scope5 settings: ActiveDisplayYMinimum=-0.57271  ActiveDisplayYMaximum=0.19884  DataLoggingVariableName=ScopeData7
      Scope6 settings: ActiveDisplayYMinimum=-0.00021  ActiveDisplayYMaximum=0.0004  DataLoggingVariableName=ScopeData4
      Scope7 settings: ActiveDisplayYMinimum=0.9  ActiveDisplayYMaximum=1.1  DataLoggingVariableName=ScopeData14
  Selector : Selector  InputPortWidth=2  IndexOptions=Index vector (dialog)  Indices=[2 1]  OutputSizes=1
  Sum : Sum  Inputs=+--+  SaturateOnIntegerOverflow=on
  Sum2 : Sum  Inputs=|++
  Sum{26,28,30,32,34,36,39,41,43} (9 alike) : Sum  Inputs=|+-  SaturateOnIntegerOverflow=on
  Sum{29,33,37..38,42,45} (6 alike) : Sum  Inputs=|++  SaturateOnIntegerOverflow=on
  Sum31 : Sum  Inputs=+++  SaturateOnIntegerOverflow=on
  Sum35 : Sum  Inputs=-+  SaturateOnIntegerOverflow=on
  Sum40 : Sum  Inputs=+++  SaturateOnIntegerOverflow=on
  Sum44 : Sum  Inputs=-+  SaturateOnIntegerOverflow=on
  Sum9 : Sum  Inputs=-+-  SaturateOnIntegerOverflow=on
  Switch2 : Switch  Criteria=u2 ~= 0  Threshold=0.5  InputSameDT=off
  Switch3 : Switch  Criteria=u2 ~= 0  Threshold=0.5  InputSameDT=off
  Terminator : Terminator
  Transport Delay{12,16,18,20,22..23} (6 alike) : TransportDelay  DelayTime=DataDelay(2,1)
  Transport Delay{13..15,17,19,21} (6 alike) : TransportDelay  DelayTime=DataDelay(4,2)
  in_D_PI : Subsystem  Commented=on  mask{KP_=0.1, KI_=0.1, Upper_limit=inf, Lower_limit=-inf, Upper_saturation_limit=inf, Lower_saturation_limit=-inf, integrator_init=Md_A_0}
      mask prompts: KP_ "比例系数P"; KI_ "积分系数I"; Upper_limit "限幅上限"; Lower_limit "限幅下限"; Upper_saturation_limit "积分饱和上限"; Lower_saturation_limit "积分饱和下限"; integrator_init "积分初始值"
      mask DialogControl Container4 Prompt: 控制参数
      mask DialogControl Container5 Prompt: 初始值
      mask Display: disp('PI')
  output : Subsystem
  w0 : Constant
  xy->dq : Subsystem
  m : Outport
  isxy : Outport  Port=2
  GBxy : Outport  Port=3
  tag scope: DWES1DT=global, Dess1=global, Dess_avg1=global, Hess1=global, Hess_avg1=global, ROCOF_ES1=global, W_ES1=global, WreES1=global, epi1=global, yita1=global
  wires:
  Selector/1 -> R_choke1/1
  Sum/1 -> Scope4/1, R_choke3/1
  R_choke3/1 -> Switch2/3
  Ground/1 -> Bistable2/2
  R_choke2/1 -> Sum/4
  R_choke/1 -> Sum/3
  [ucxy] -> Sum/2
  output/1(m) -> m/1
  NOT/1 -> " control1"/Enable
  R_choke1/1 -> R_choke2/1
  Bistable2/1 -> NOT/1, [outage]
  Isxy/1 -> Switch3/3
  [isxy] -> xy->dq/1(Ixy)
  [isxy] -> output/1(is_xy)
  output/2(isxy) -> isxy/1
  [xy_dq_delta] -> " control1"/3(delta)
  xy->dq/1(Idq) -> [isdq], Scope/1
  Bistable2/2 -> Terminator/1
  outage/1 -> Bistable2/1
  [outage] -> Switch2/2, Switch3/2
  [isdq] -> " control1"/2(isdq)
  " control1"/1(ucx) -> Mux/1
  Switch2/1 -> Isxy/1
  Switch3/1 -> R_choke/1, Selector/1, [isxy]
  Mux/1 -> Scope12/1, [ucxy]
  [usdq] -> " control1"/1(usdq)
  output/3(GBxy) -> GBxy/1
  Constant1/1 -> Switch2/1, Switch3/1
  " control1"/2(ucy) -> Mux/2
  [usdq] -> Product2/1
  Add1/1 -> Scope5/1, output/2(Pe)  "Pess1"
  Product2/1 -> Add1/1
  [isdq] -> Product2/2
  Product1/1 -> Scope6/1, [DWES1DT], Int2/1
  Sum26/1 -> [WreES1], Product4/2, Gain1/1
  Int2/1 -> Sum26/1
  w0/1 -> Sum26/2
  Sum9/1 -> Product1/1, Scope11/1
  Constant/1 -> Divide/1
  Divide/1 -> Product1/2, Scope7/1
  [Hess1] -> Divide/2
  us_xy/1 -> Mux4/1, Sum/1
  Fcn3/1 -> Mux3/1
  Fcn4/1 -> Mux3/2
  Mux4/1 -> Fcn3/1, Fcn4/1
  [xy_dq_delta] -> Mux4/2, xy->dq/2(Theta)
  Mux3/1 -> Scope3/1, [usdq]
  Gain4/1 -> Sum9/3
  Product4/1 -> Sum9/1
  Int1/1 -> Scope13/1, [xy_dq_delta]
  Add2/1 -> Gain4/1, Scope10/1  "Pess1"
  [usdq] -> Product3/1
  [isdq] -> Product3/2
  Product3/1 -> Add2/1
  Transport Delay19/1 -> [Davg4rec]
  R_choke20/1 -> Sum31/2
  R_choke19/1 -> Sum31/1
  [Dess_avg1] -> Sum28/1
  Transport Delay13/1 -> Mux5/2
  Transport Delay12/1 -> Mux5/1
  [Dess_avg1] -> Sum30/1
  Mux6/1 -> [W_ES1]  "W_ES1"
  [WreES1] -> Mux6/3  "W1"
  Sum38/1 -> [Hess1]  "Hess1"
  Constant5/1 -> Sum45/1
  Sum45/1 -> Scope15/1, [Dess1]  "Dess1"
  Constant6/1 -> Sum38/1
  [epi1] -> Sum34/1
  R_choke21/1 -> Sum31/3
  Integrator6/1 -> [epi1]
  Sum35/1 -> R_choke21/1
  Sum31/1 -> Integrator7/1
  Integrator7/1 -> [Dess_avg1], Scope14/1, Sum35/1
  Transport Delay21/1 -> [epi4rec]
  [epi2] -> Transport Delay20/1
  [epi4rec] -> Sum34/2
  [DWES1DT] -> Mux5/3  "df1dt"
  [Davg4rec] -> Sum30/2
  [yita2rec] -> Sum41/2
  [yita1] -> Sum41/1
  Sum40/1 -> Integrator9/1
  [deltaDess1] -> Sum45/2, Gain/1
  R_choke18/1 -> Integrator6/1
  [Havg4rec] -> Sum39/2
  [epi1] -> Sum32/1
  [Havg2rec] -> Sum36/2
  Sum42/1 -> R_choke16/1
  [Dess_avg2] -> Transport Delay18/1
  Transport Delay20/1 -> [epi2rec]
  Transport Delay14/1 -> [Havg4rec]
  [Hess_avg1] -> Sum39/1
  Mux5/1 -> [ROCOF_ES1]  "ROCOF_ES1"
  Integrator9/1 -> [Hess_avg1], Sum44/1
  Sum29/1 -> R_choke19/1, R_choke18/1
  [Davg2rec] -> Sum28/2
  [yita2] -> Transport Delay23/1
  Sum37/1 -> R_choke15/1, R_choke14/1
  R_choke14/1 -> Integrator8/1
  Integrator8/1 -> [yita1]
  Transport Delay18/1 -> [Davg2rec]
  R_choke17/1 -> Sum40/3
  Transport Delay17/1 -> Mux6/2
  R_choke15/1 -> Sum40/1
  R_choke16/1 -> Sum40/2
  [Hess_avg1] -> Sum36/1
  [deltaHess1] -> Sum38/2, Gain2/1
  Sum44/1 -> R_choke17/1
  Sum33/1 -> R_choke20/1
  Transport Delay23/1 -> [yita2rec]
  Transport Delay16/1 -> Mux6/1
  [epi2rec] -> Sum32/2
  Transport Delay22/1 -> [Havg2rec]
  Transport Delay15/1 -> [yita4rec]
  [Hess_avg2] -> Transport Delay22/1
  [Dess1] -> Product4/1
  Gain1/1 -> Int1/1
  [yita4rec] -> Sum43/2
  [yita1] -> Sum43/1
  Gain/1 -> Sum35/2
  Gain2/1 -> Sum44/2
  [Dess_avg4] -> Transport Delay19/1
  [epi4] -> Transport Delay21/1
  [Hess_avg4] -> Transport Delay14/1
  [yita4] -> Transport Delay15/1
  [WreES2] -> Gain12/1  "W2"
  Gain12/1 -> Transport Delay16/1
  [WreES4] -> Gain13/1  "W4"
  Gain13/1 -> Transport Delay17/1
  [DWES2DT] -> Gain14/1  "df2dt"
  Gain14/1 -> Transport Delay12/1
  [DWES4DT] -> Gain15/1  "df4dt"
  Gain15/1 -> Transport Delay13/1
  Gain3/1 -> Sum29/1
  Sum28/1 -> Gain3/1
  Gain5/1 -> Sum33/1
  Sum32/1 -> Gain5/1
  Sum36/1 -> Gain6/1
  Gain6/1 -> Sum37/1
  Gain7/1 -> Sum42/1
  Sum41/1 -> Gain7/1
  Sum30/1 -> Gain8/1
  Gain8/1 -> Sum29/2
  Sum34/1 -> Gain9/1
  Gain9/1 -> Sum33/2
  Sum39/1 -> Gain10/1
  Gain10/1 -> Sum37/2
  Sum43/1 -> Gain11/1
  Gain11/1 -> Sum42/2
  [deltapes1] -> Sum2/1
  Sum2/1 -> [Pref]
  Constant3/1 -> Sum2/2
  [Pref] -> Sum9/2
  Divide2/1 -> Gain17/1
  Constant4/1 -> Divide2/2
  From9/1 -> Divide2/1
  in_D_PI/1(Out1) -> Goto9/1
  Gain17/1 -> in_D_PI/1(In1)
